simulink model "Path2SetPoint"  (R2015b)
settings: Solver=FixedStepAuto  StartTime=0.0  StopTime=inf  FixedStep=0.05  RelTol=1e-3
model workspace (MAT data in the model file):
  SL_ROS_VariableLengthArrays_MaxSizes.CommonInfo.ArrayTruncateAction = 'EmitWarning'
  SL_ROS_VariableLengthArrays_MaxSizes.MsgTypeMap = containers.Map
  SL_ROS_VariableLengthArrays_MaxSizes.MsgTypeMap.serialization.keys = {'std_msgs/Float32MultiArray'}
  SL_ROS_VariableLengthArrays_MaxSizes.MsgTypeMap.serialization.values{1}.PropertyName = 'Data'
  SL_ROS_VariableLengthArrays_MaxSizes.MsgTypeMap.serialization.values{1}.DataType = 'single'
  SL_ROS_VariableLengthArrays_MaxSizes.MsgTypeMap.serialization.values{1}.MaxLength = 256
  SL_ROS_VariableLengthArrays_MaxSizes.MsgTypeMap.serialization.uniformity = 0
  SL_ROS_VariableLengthArrays_MaxSizes.MsgTypeMap.serialization.keyType = 'char'
  SL_ROS_VariableLengthArrays_MaxSizes.MsgTypeMap.serialization.valueType = 'any'
undefined symbols (not defined in the file or in its folder): X, Y, Z
libraries: robotlib x11, realtime_pacer_lib x1
settings Model: Creator=einar  LastModifiedBy=saucer
settings OptimizationCC: OptimizeModelRefInitCode=on  LifeSpan=Inf  MaxStackSize=64
settings HardwareCC: ProdBitPerPointer=32  ProdLargestAtomicFloat=None  ProdIntDivRoundTo=Undefined  ProdEndianess=Unspecified  ProdWordSize=32  ProdHWDeviceType=Generic->Unspecified (assume 32-bit Generic)
settings RTWCC: SystemTargetFile=ert.tlc  TemplateMakefile=ert_default_tmf  Description=Embedded Coder  Toolchain=Catkin  TargetLang=C++
settings CodeAppCC: IgnoreCustomStorageClasses=off
settings ERTTargetCC: SupportContinuousTime=on  SupportVariableSizeSignals=on

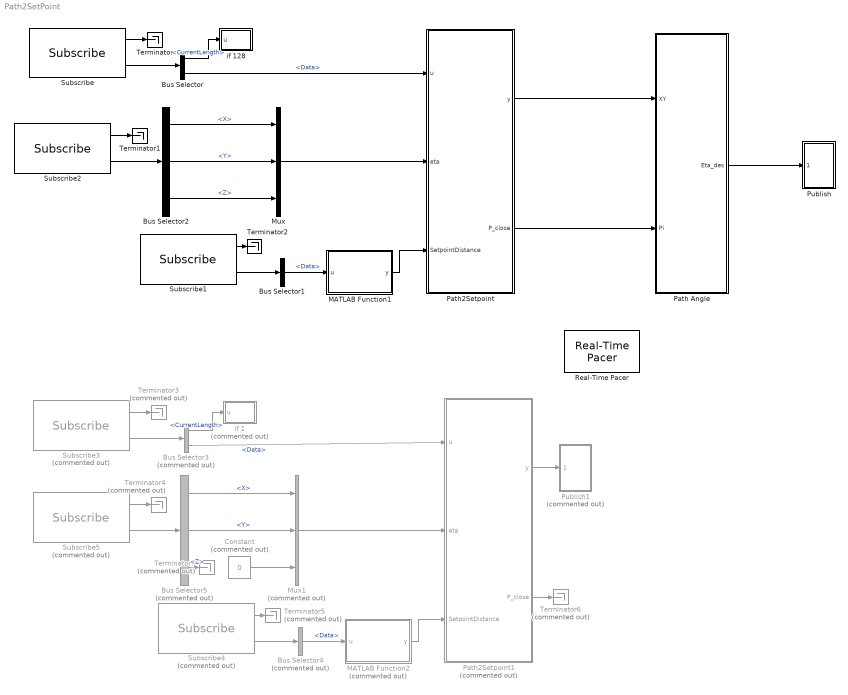
== system Path2SetPoint ==
  Bus Selector : BusSelector  OutputSignals=Data_SL_Info.CurrentLength,Data
  Bus Selector1 : BusSelector  OutputSignals=Data
  Bus Selector2 : BusSelector  OutputSignals=X,Y,Z
  Bus Selector3 : BusSelector  Commented=on  OutputSignals=Data_SL_Info.CurrentLength,Data
  Bus Selector4 : BusSelector  Commented=on  OutputSignals=Data
  Bus Selector5 : BusSelector  Commented=on  OutputSignals=X,Y,Z
  Constant : Constant  Commented=on  Value=0
  MATLAB Function1 : MATLAB Function  TreatAsAtomicUnit=on
  MATLAB Function2 : MATLAB Function  Commented=on  TreatAsAtomicUnit=on
  Mux : Mux  Inputs=3
  Mux1 : Mux  Commented=on  Inputs=3
  Path Angle : Subsystem
  Path2Setpoint : MATLAB Function  TreatAsAtomicUnit=on
  Path2Setpoint1 : MATLAB Function  Commented=on  TreatAsAtomicUnit=on
  Publish : Subsystem
  Publish1 : Subsystem  Commented=on
  Real-Time Pacer : realtime_pacer_lib/Real-Time Pacer  simTimePerRealTime=1
  Subscribe : robotlib/Subscribe  SourceLibraryInfo=This block requires Robotics System Toolbox  topicSource=Specify your own  topic=/Path  messageType=std_msgs/Float32MultiArray  sampleTime=-1  messageQueueLength=1
  Subscribe1 : robotlib/Subscribe  SourceLibraryInfo=This block requires Robotics System Toolbox  topicSource=Specify your own  topic=/SetPointDist  messageType=std_msgs/Float64  sampleTime=-1  messageQueueLength=1
  Subscribe2 : robotlib/Subscribe  SourceLibraryInfo=This block requires Robotics System Toolbox  topicSource=Specify your own  topic=/Position  messageType=geometry_msgs/Vector3  sampleTime=-1  messageQueueLength=1
  Subscribe3 : robotlib/Subscribe  Commented=on  SourceLibraryInfo=This block requires Robotics System Toolbox  topicSource=Specify your own  topic=/Path  messageType=std_msgs/Float32MultiArray  sampleTime=-1  messageQueueLength=1
  Subscribe4 : robotlib/Subscribe  Commented=on  SourceLibraryInfo=This block requires Robotics System Toolbox  topicSource=Specify your own  topic=/SetPointDist  messageType=std_msgs/Float64  sampleTime=-1  messageQueueLength=1
  Subscribe5 : robotlib/Subscribe  Commented=on  SourceLibraryInfo=This block requires Robotics System Toolbox  topicSource=Specify your own  topic=/Position  messageType=geometry_msgs/Vector3  sampleTime=-1  messageQueueLength=1
  Terminator : Terminator
  Terminator1 : Terminator
  Terminator2 : Terminator
  Terminator{3..7} (5 alike) : Terminator  Commented=on
  if 1 : MATLAB Function  Commented=on  TreatAsAtomicUnit=on
  if 128 : MATLAB Function  TreatAsAtomicUnit=on
  wires:
  Subscribe/2 -> Bus Selector/1
  Bus Selector/2 -> Path2Setpoint/1(u)  "<Data>"
  Mux/1 -> Path2Setpoint/2(eta)
  MATLAB Function1/1(y) -> Path2Setpoint/3(SetpointDistance)
  Subscribe1/2 -> Bus Selector1/1
  Bus Selector1/1 -> MATLAB Function1/1(u)  "<Data>"
  Bus Selector2/1 -> Mux/1  "<X>"
  Subscribe2/2 -> Bus Selector2/1
  Bus Selector2/2 -> Mux/2  "<Y>"
  Bus Selector/1 -> if 128/1(u)  "<CurrentLength>"
  Subscribe/1 -> Terminator/1
  Subscribe2/1 -> Terminator1/1
  Bus Selector2/3 -> Mux/3  "<Z>"
  Subscribe1/1 -> Terminator2/1
  Path2Setpoint/2(P_close) -> Path Angle/2(Pi)
  Path Angle/1(Eta_des) -> Publish/1(SetPoint)
  Path2Setpoint/1(y) -> Path Angle/1(XY)
  Subscribe3/2 -> Bus Selector3/1
  Bus Selector3/2 -> Path2Setpoint1/1(u)  "<Data>"
  Mux1/1 -> Path2Setpoint1/2(eta)
  MATLAB Function2/1(y) -> Path2Setpoint1/3(SetpointDistance)
  Subscribe4/2 -> Bus Selector4/1
  Bus Selector4/1 -> MATLAB Function2/1(u)  "<Data>"
  Bus Selector5/1 -> Mux1/1  "<X>"
  Subscribe5/2 -> Bus Selector5/1
  Bus Selector5/2 -> Mux1/2  "<Y>"
  Bus Selector3/1 -> if 1/1(u)  "<CurrentLength>"
  Subscribe3/1 -> Terminator3/1
  Subscribe5/1 -> Terminator4/1
  Subscribe4/1 -> Terminator5/1
  Path2Setpoint1/2(P_close) -> Terminator6/1
  Path2Setpoint1/1(y) -> Publish1/1(SetPoint)
  Constant/1 -> Mux1/3
  Bus Selector5/3 -> Terminator7/1  "<Z>"

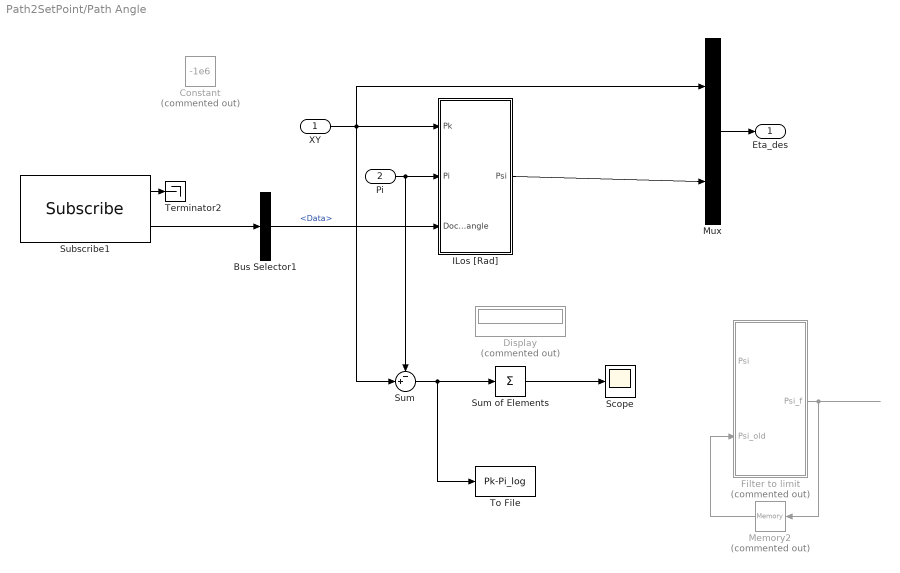
== system Path2SetPoint/Path Angle ==
  XY : Inport
  Pi : Inport  Port=2
  Bus Selector1 : BusSelector  OutputSignals=Data
  Constant : Constant  Commented=on  Value=-1e6
  Display : Display  Commented=on
  Filter to limit : MATLAB Function  Commented=on  TreatAsAtomicUnit=on
  ILos [Rad] : MATLAB Function  TreatAsAtomicUnit=on
  Memory2 : Memory  Commented=on  InheritSampleTime=on
  Mux : Mux  Inputs=2
  Scope : Scope
  Subscribe1 : robotlib/Subscribe  SourceLibraryInfo=This block requires Robotics System Toolbox  topicSource=Select from ROS network  topic=/Docking_heading  messageType=std_msgs/Float64  sampleTime=-1  messageQueueLength=1
  Sum : Sum  Inputs=-+|
  Sum of Elements : Sum  Inputs=+
  Terminator2 : Terminator
  To File : ToFile  Filename=Pk-Pi_log  SaveFormat=Timeseries
  Eta_des : Outport
  wires:
  XY/1 -> Sum/2, Mux/1, ILos [Rad]/1(Pk)
  Pi/1 -> Sum/1, ILos [Rad]/2(Pi)
  Mux/1 -> Eta_des/1
  ILos [Rad]/1(Psi) -> Mux/2
  Sum/1 -> Sum of Elements/1, To File/1
  Sum of Elements/1 -> Scope/1
  Filter to limit/1(Psi_f) -> Memory2/1
  Memory2/1 -> Filter to limit/2(Psi_old)
  Subscribe1/2 -> Bus Selector1/1
  Subscribe1/1 -> Terminator2/1
  Bus Selector1/1 -> ILos [Rad]/3(Docking_angle)  "<Data>"

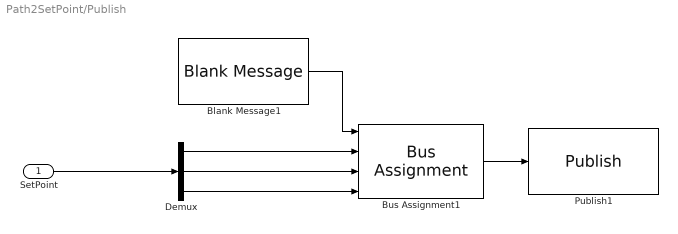
== system Path2SetPoint/Publish ==
  SetPoint : Inport
  Blank Message1 : robotlib/Blank Message  SourceLibraryInfo=This block requires Robotics System Toolbox  messageType=geometry_msgs/Vector3  SampleTime=inf
  Bus Assignment1 : BusAssignment  AssignedSignals=X,Y,Z
  Demux : Demux  Outputs=3
  Publish1 : robotlib/Publish  SourceLibraryInfo=This block requires Robotics System Toolbox  topicSource=Specify your own  topic=/SetPoint  messageType=geometry_msgs/Vector3  messageQueueLength=1
  wires:
  Demux/2 -> Bus Assignment1/3
  Demux/1 -> Bus Assignment1/2
  SetPoint/1 -> Demux/1
  Bus Assignment1/1 -> Publish1/1
  Demux/3 -> Bus Assignment1/4
  Blank Message1/1 -> Bus Assignment1/1

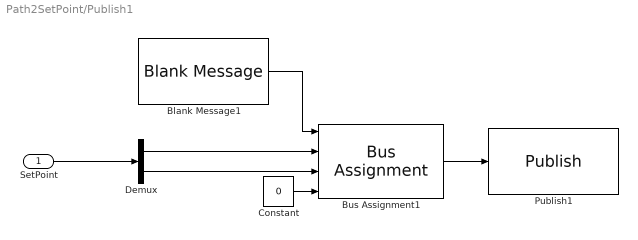
== system Path2SetPoint/Publish1 ==
  SetPoint : Inport
  Blank Message1 : robotlib/Blank Message  SourceLibraryInfo=This block requires Robotics System Toolbox  messageType=geometry_msgs/Vector3  SampleTime=inf
  Bus Assignment1 : BusAssignment  AssignedSignals=X,Y,Z
  Constant : Constant  Value=0
  Demux : Demux  Outputs=2
  Publish1 : robotlib/Publish  SourceLibraryInfo=This block requires Robotics System Toolbox  topicSource=Specify your own  topic=/SetPoint  messageType=geometry_msgs/Vector3  messageQueueLength=1
  wires:
  Demux/2 -> Bus Assignment1/3
  Demux/1 -> Bus Assignment1/2
  SetPoint/1 -> Demux/1
  Bus Assignment1/1 -> Publish1/1
  Blank Message1/1 -> Bus Assignment1/1
  Constant/1 -> Bus Assignment1/4

== matlab function Path2SetPoint/if 128 ==
  data: u input
function fcn(u)
if u==128
    error('Length set to %i. Must be 256! See Tool -> ROS -> Manage Array Sizes. Float32MultiArray Must have length 256',u)
end
end

== matlab function Path2SetPoint/MATLAB Function2 ==
  data: u input; y output
function y = fcn(u)

    y=u;    

if u==0
    %y(1)=0.25;
    y(1)=0.2;
end
end

== matlab function Path2SetPoint/Path2Setpoint ==
  data: u input; y output; eta input; SetpointDistance input; P_close output
function [y,P_close] = fcn(u,eta,SetpointDistance)
%Generates setpoint based on path, setpointdistance and position
y=[0; 0];
Z=length(u);
eta=eta(1:2);

%#codegen
%save('TESTlist2Eta') 
Values=[u(1:Z/2) u(Z/2+1:end)];

Iterate2=min([find(Values==1000) ;size(Values,1)]);
e= 0;
P_close = [0;0];
if u(1,1)==0&&sum((u==0))==Z;
    y=[0; 0];
elseif Iterate2==2
    %    asl=1
    %    a=asl(2);
    y(1)=Values(1,2);
    y(2)=Values(1,1);
else
    %DiscretizedPath
    DiscretizedStep=0.01;
    counter=1;
    DiscretizedPath=zeros(5000,2);
    for k=2:Iterate2-1
        DistanceTraveled=norm([Values(k,1)-Values(k-1,1) Values(k,2)-Values(k-1,2)]) ;
        DistanceTraveledX=Values(k,1)-Values(k-1,1);
        DistanceTraveledY=Values(k,2)-Values(k-1,2);
        Niterations=floor(DistanceTraveled/DiscretizedStep);
        for z=1:Niterations
            DiscretizedPath(counter,1)=Values(k-1,1)+z*DistanceTraveledX/Niterations;
            DiscretizedPath(counter,2)=Values(k-1,2)+z*DistanceTraveledY/Niterations;
        counter=counter+1;
        end
    end
    DiscretizedEnds=min([find(DiscretizedPath==inf) ;size(DiscretizedPath,1)]);
    DiscretizedPath=DiscretizedPath(1:DiscretizedEnds-1,1:2);

    eta=eta(2:-1:1)';



    %NearestPointPos=4;
    %AvstandSaved=1000;
    %for i=1:64


    [Avstand, NearestPointPos]=min((sum((abs(DiscretizedPath-repmat(eta,size(DiscretizedPath,1),1))).^2')));
    P_close(1) = DiscretizedPath(NearestPointPos,2);
    P_close(2) = DiscretizedPath(NearestPointPos,1);
    %e=Avstand; 
%     if (NearestPointPos-3)>1
%         SetPoint=NearestPointPos-3;
% 
%     else
%         SetPoint=1;
%     end
    NIter=round(SetpointDistance/DiscretizedStep);

    SetPoint=max([1 NearestPointPos-NIter]);
    y(1)=DiscretizedPath(SetPoint,2);
    y(2)=DiscretizedPath(SetPoint,1);

end
end

== matlab function Path2SetPoint/MATLAB Function1 ==
  data: u input; y output
function y = fcn(u)

    y=u;    

if u==0
    %y(1)=0.25;
    y(1)=0.2;
end
end

== matlab function Path2SetPoint/Path Angle/ILos [Rad] ==
  data: Pk input; Pi input; Psi output; Docking_angle input
function Psi = Path_angle(Pk,Pi,Docking_angle)
    if Docking_angle ~= -1e6
        disp('Huston we are Docking!')
        Psi = Docking_angle;
    else
        alpha = atan2(Pk(2)-Pi(2),Pk(1)-Pi(1));
        %alpha = atan2(Pk(1)-Pi(1),Pk(2)-Pi(2));
        Psi = alpha;
    end
end

== matlab function Path2SetPoint/Path Angle/Filter to limit ==
  data: Psi input; Psi_old input; Psi_f output; psi_d_max parameter
function Psi_f = Analog_filter(Psi,Psi_old,psi_d_max)
    if abs(Psi-Psi_old) > psi_d_max*pi/180;
        Psi_f = Psi_old +  psi_d_max*pi/180*sign(Psi-Psi_old);
    else
        Psi_f = Psi;
    end
    
end

== matlab function Path2SetPoint/Path2Setpoint1 ==
  data: u input; y output; eta input; SetpointDistance input; P_close output
function [y,P_close] = fcn(u,eta,SetpointDistance)
%Generates setpoint based on path, setpointdistance and position
y=[0; 0];
Z=length(u);
eta=eta(1:2);

%#codegen
%save('TESTlist2Eta') 
Values=[u(1:Z/2) u(Z/2+1:end)];

Iterate2=min([find(Values==1000) ;size(Values,1)]);
e= 0;
P_close = [0;0];
if u(1,1)==0&&sum((u==0))==Z;
    y=[0; 0];
elseif Iterate2==2
    %    asl=1
    %    a=asl(2);
    y(1)=Values(1,2);
    y(2)=Values(1,1);
else
    %DiscretizedPath
    DiscretizedStep=0.01;
    counter=1;
    DiscretizedPath=zeros(5000,2);
    for k=2:Iterate2-1
        DistanceTraveled=norm([Values(k,1)-Values(k-1,1) Values(k,2)-Values(k-1,2)]) ;
        DistanceTraveledX=Values(k,1)-Values(k-1,1);
        DistanceTraveledY=Values(k,2)-Values(k-1,2);
        Niterations=floor(DistanceTraveled/DiscretizedStep);
        for z=1:Niterations
            DiscretizedPath(counter,1)=Values(k-1,1)+z*DistanceTraveledX/Niterations;
            DiscretizedPath(counter,2)=Values(k-1,2)+z*DistanceTraveledY/Niterations;
        counter=counter+1;
        end
    end
    DiscretizedEnds=min([find(DiscretizedPath==inf) ;size(DiscretizedPath,1)]);
    DiscretizedPath=DiscretizedPath(1:DiscretizedEnds-1,1:2);

    eta=eta(2:-1:1)';



    %NearestPointPos=4;
    %AvstandSaved=1000;
    %for i=1:64


    [Avstand, NearestPointPos]=min((sum((abs(DiscretizedPath-repmat(eta,size(DiscretizedPath,1),1))).^2')));
    P_close(1) = DiscretizedPath(NearestPointPos,2);
    P_close(2) = DiscretizedPath(NearestPointPos,1);
    %e=Avstand; 
%     if (NearestPointPos-3)>1
%         SetPoint=NearestPointPos-3;
% 
%     else
%         SetPoint=1;
%     end
    NIter=round(SetpointDistance/DiscretizedStep);

    SetPoint=max([1 NearestPointPos-NIter]);
    y(1)=DiscretizedPath(SetPoint,2);
    y(2)=DiscretizedPath(SetPoint,1);

end
end

== matlab function Path2SetPoint/if 1 ==
  data: u input
function fcn(u)
if u==128
    error('Length set to %i. Must be 256! See Tool -> ROS -> Manage Array Sizes. Float32MultiArray Must have length 256',u)
end
end
